simulink model "VoltageSourceSimulation"  (Simulink 8.6)
settings: Solver=VariableStepAuto  StartTime=0.0  StopTime=0.0001  RelTol=1e-3
values from neighbouring files (symbols this model uses):
  c2_val = 0.1e-6    (= 1e-07)    [VoltageSourceController.m]
  l2_val = 0.01e-6    (= 1e-08)    [VoltageSourceController.m]
  rc2_val = 0.0001    [VoltageSourceController.m]
  rl2_val = 0.0001    [VoltageSourceController.m]
  Vd_val = 100    [CurrentSourceController.m]    (also in VoltageSourceController.m)
undefined symbols (not defined in the file or in its folder): den_c2, num_c2
libraries: powerlib x9, powerlib_meascontrol x1
settings Model: Creator=Akshay  LastModifiedBy=Akshay
settings SolverCC: ZeroCrossAlgorithm=Adaptive
settings DataIOCC: SaveFormat=Dataset  SignalLoggingSaveFormat=Dataset
settings OptimizationCC: ExpressionDepthLimit=128
settings DebuggingCC: UnderspecifiedInitializationDetection=Simplified  MergeDetectMultiDrivingBlocksExec=error  SolverPrmCheckMsg=none  FcnCallInpInsideContextMsg=EnableAllAsError  StateNameClashWarn=none
settings HardwareCC: ProdBitPerPointer=64  ProdLargestAtomicFloat=Float  ProdIntDivRoundTo=Zero  ProdEndianess=LittleEndian  ProdWordSize=64  ProdHWDeviceType=Intel->x86-64 (Windows64)
settings GRTTargetCC: GeneratePreprocessorConditionals=Use local settings  CombineOutputUpdateFcns=on  GRTInterface=off
settings ConfigComp: CovModelRefEnable=off

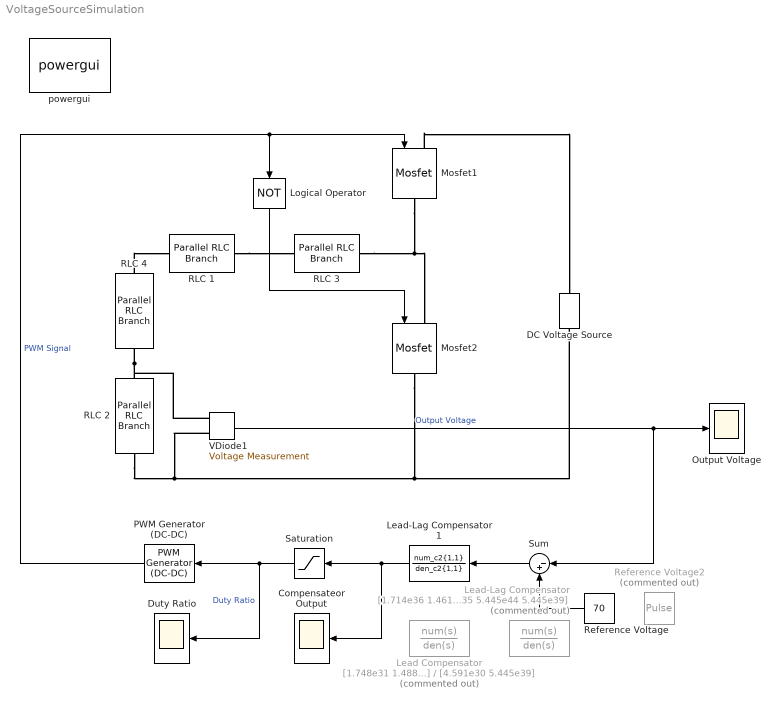
== system VoltageSourceSimulation ==
  " RLC 1" : powerlib/Elements/Parallel RLC Branch  LConnTagsString=a  RConnTagsString=__new0  BranchType=R  Resistance=rl2_val  Inductance=5e-6  SetiL0=off  InitialCurrent=0  Capacitance=0.3e-6  Setx0=off  InitialVoltage=0  Measurements=None
  " RLC 2" : powerlib/Elements/Parallel RLC Branch  LConnTagsString=a  RConnTagsString=__new0  BranchType=C  Resistance=1  Inductance=1e-3  SetiL0=off  InitialCurrent=0  Capacitance=c2_val  Setx0=off  InitialVoltage=50  Measurements=None
  " RLC 3" : powerlib/Elements/Parallel RLC Branch  LConnTagsString=a  RConnTagsString=__new0  BranchType=L  Resistance=50  Inductance=l2_val  SetiL0=off  InitialCurrent=0  Capacitance=0.3e-6  Setx0=off  InitialVoltage=0  Measurements=None
  " RLC 4" : powerlib/Elements/Parallel RLC Branch  LConnTagsString=a  RConnTagsString=__new0  BranchType=R  Resistance=rc2_val  Inductance=1e-3  SetiL0=off  InitialCurrent=0  Capacitance=0.1e-6  Setx0=off  InitialVoltage=0  Measurements=None
  Compensateor Output : Scope
  DC Voltage Source : powerlib/Electrical Sources/DC Voltage Source  Amplitude=Vd_val  Measurements=Voltage
  Duty Ratio : Scope
  Lead Compensator : TransferFcn  Commented=on  Numerator=[1.748e31 1.488e39]  Denominator=[4.591e30 5.445e39]
  Lead-Lag Compensator : TransferFcn  Commented=on  Numerator=[1.714e36 1.461e44 1.459e49]  Denominator=[4.591e35 5.445e44 5.445e39]
  Lead-Lag Compensator1 : TransferFcn  Numerator=num_c2{1,1}  Denominator=den_c2{1,1}
  Logical Operator : Logic  Operator=NOT  AllPortsSameDT=off  OutDataTypeStr=boolean
  Mosfet1 : powerlib/Power Electronics/Mosfet  Ron=0.00001  Lon=0  Rd=0.0000000000001  Vfd=0  IC=0  Rs=1e5  Cs=inf  Measurements=off
  Mosfet2 : powerlib/Power Electronics/Mosfet  Ron=0.00001  Lon=0  Rd=0.0000000000001  Vfd=0  IC=0  Rs=1e5  Cs=inf  Measurements=off
  Output Voltage : Scope
  PWM Generator (DC-DC) : powerlib_meascontrol/Pulse & Signal Generators/PWM Generator (DC-DC)  Fsw=1e6  Ts=0
  Reference Voltage : Constant  Value=70
  Reference Voltage2 : DiscretePulseGenerator  Commented=on  PulseType=Time based  Amplitude=70  Period=180e-6  PulseWidth=6
  Saturation : Saturate  UpperLimit=1  LowerLimit=0  ZeroCross=off
  Sum : Sum  Inputs=|-+
  VDiode1 : powerlib/Measurements/Voltage Measurement  PhasorSimulation=off  OutputType=Complex  PSBequivalent=0
  powergui : powerlib/powergui  Priority=1  SimulationMode=Continuous  SolverType=Backward Euler  SampleTime=5e-07  frequency=60  SPID=on  DisableSnubberDevices=off  DisableRonSwitches=off  DisableVfSwitches=off  SwTol=0  DisplayEquations=off  Interpol=off  ExternalGateDelay=off  methode=off  Ts=0  FunctionMessages=off  echomessages=off  HookPort=off  EnableUseOfTLC=off  x0status=zero  frequencyindice=0  Pbase=100e6  ErrMax=1e-4  Iterations=50  UnitsV=kV  UnitsW=MW  buscounter=0  RestoreLinks=warning  ResistiveCurrentMeasurement=off  Frange=[0:2:500]  Ylog=off  Xlog=on  ShowGrid=off  save=off  variable=ZData  structure=ScopeData  ZoomFFT=off  StartTime=0.0  cycles=5  DisplayStyle=2  fundamental=50  FreqAxis=off  MaxFrequency=50000  frequencyindicesteady=1  RmsSteady=1  display=off
  wires:
  Logical Operator/1 -> Mosfet2/1
  VDiode1/1 -> Output Voltage/1, Sum/1  "Output Voltage"
  Sum/1 -> Lead-Lag Compensator1/1
  Saturation/1 -> Duty Ratio/1, PWM Generator (DC-DC)/1  "Duty Ratio"
  PWM Generator (DC-DC)/1 -> Mosfet1/1, Logical Operator/1  "PWM Signal"
  Reference Voltage/1 -> Sum/2
  Lead-Lag Compensator1/1 -> Compensateor Output/1, Saturation/1
  connections:
  Mosfet1/RConn1 -- " RLC 3"/RConn1 -- Mosfet2/LConn1
  Mosfet1/LConn1 -- DC Voltage Source/RConn1
  DC Voltage Source/LConn1 -- " RLC 2"/RConn1 -- VDiode1/LConn2 -- Mosfet2/RConn1
  " RLC 1"/RConn1 -- " RLC 3"/LConn1
  " RLC 2"/LConn1 -- VDiode1/LConn1 -- " RLC 4"/RConn1
  " RLC 4"/LConn1 -- " RLC 1"/LConn1
